simulink model "Pendulo_fuzzy_control"  (R2016a)
settings: Solver=VariableStepAuto  StartTime=0.0  StopTime=10.0  RelTol=1e-3
undefined symbols (not defined in the file or in its folder): Pendulo_fuzzy_logic
libraries: fuzblock x1
settings Model: Creator=Daniel  LastModifiedBy=Daniel

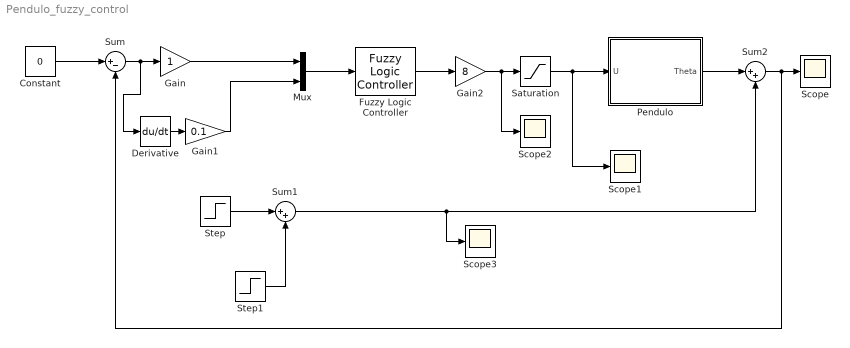
== system Pendulo_fuzzy_control ==
  Constant : Constant  Value=0
  Derivative : Derivative
  Fuzzy Logic Controller : fuzblock/Fuzzy Logic  Controller  fis=[Pendulo_fuzzy_logic]
  Gain : Gain
  Gain1 : Gain  Gain=0.1
  Gain2 : Gain  Gain=8
  Mux : Mux  Inputs=2
  Pendulo : Subsystem
  Saturation : Saturate  UpperLimit=10  LowerLimit=-10
  Scope{,1..3} (4 alike) : Scope
  Step : Step  Time=4  After=0.2  SampleTime=0
  Step1 : Step  Time=5  After=-0.2  SampleTime=0
  Sum : Sum  Inputs=|+-
  Sum1 : Sum  Inputs=|++
  Sum2 : Sum  Inputs=|++
  wires:
  Sum/1 -> Derivative/1, Gain/1
  Constant/1 -> Sum/1
  Gain/1 -> Mux/1
  Gain1/1 -> Mux/2
  Step/1 -> Sum1/1
  Step1/1 -> Sum1/2
  Pendulo/1(Theta) -> Sum2/1
  Sum1/1 -> Scope3/1, Sum2/2
  Gain2/1 -> Scope2/1, Saturation/1
  Saturation/1 -> Scope1/1, Pendulo/1(U)
  Sum2/1 -> Sum/2, Scope/1
  Mux/1 -> Fuzzy Logic Controller/1
  Fuzzy Logic Controller/1 -> Gain2/1
  Derivative/1 -> Gain1/1

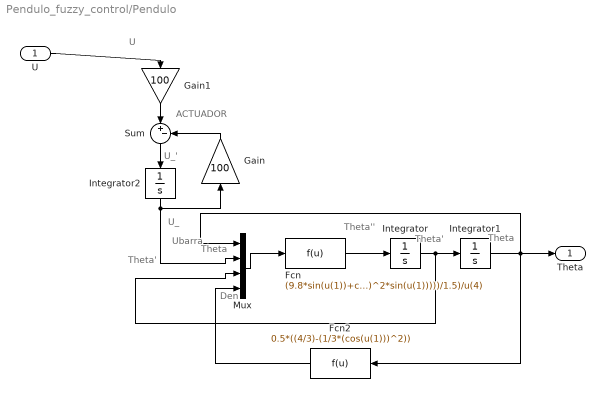
== system Pendulo_fuzzy_control/Pendulo ==
  note: Theta'
  note: Theta
  note: Theta''
  note: Theta
  note: U
  note: Ubarra
  note: Theta'
  note: Den
  note: U_'
  note: U_
  note: ACTUADOR
  U : Inport
  Fcn : Fcn  Expr=(9.8*sin(u(1))+cos(u(1))*(((-u(2)-0.25*u(3)^2*sin(u(1)))))/1.5)/u(4)
  Fcn2 : Fcn  Expr=0.5*((4/3)-(1/3*(cos(u(1)))^2))
  Gain : Gain  Gain=100  SaturateOnIntegerOverflow=on  OutDataTypeStr=Inherit: Same as input  ParamDataTypeStr=Inherit: Same as input
  Gain1 : Gain  Gain=100  SaturateOnIntegerOverflow=on  OutDataTypeStr=Inherit: Same as input  ParamDataTypeStr=Inherit: Same as input
  Integrator : Integrator
  Integrator1 : Integrator  InitialCondition=0.1
  Integrator2 : Integrator  InitialCondition=0.01
  Mux : Mux
  Sum : Sum  Inputs=|+-  SaturateOnIntegerOverflow=on  InputSameDT=on  OutDataTypeStr=Inherit: Same as first input
  Theta : Outport
  wires:
  Fcn/1 -> Integrator/1
  Mux/1 -> Fcn/1
  Integrator/1 -> Integrator1/1, Mux/3
  Integrator1/1 -> Mux/1, Theta/1, Fcn2/1
  Integrator2/1 -> Gain/1, Mux/2
  Sum/1 -> Integrator2/1
  Gain1/1 -> Sum/1
  Gain/1 -> Sum/2
  U/1 -> Gain1/1
  Fcn2/1 -> Mux/4
